simulink model "Roteiro1_Planta"  (R2019a)
settings: Solver=FixedStepAuto  StartTime=0.0  StopTime=250  FixedStep=0.1  RelTol=1e-3
values from neighbouring files (symbols this model uses):
  K = 0.4725    [Roteiro1_PlantaTermica.m]
  Kp = T/(K*L)    (= 21.164021164)    [Roteiro1_PlantaTermica.m]
  L = 10    [Roteiro1_PlantaTermica.m]
  T = 100    [Roteiro1_PlantaTermica.m]
  theta_AMB = 33.6    [Roteiro1_PlantaTermica.m]
settings Model: Creator=JoaoG-PC  LastModifiedBy=JoaoG-PC

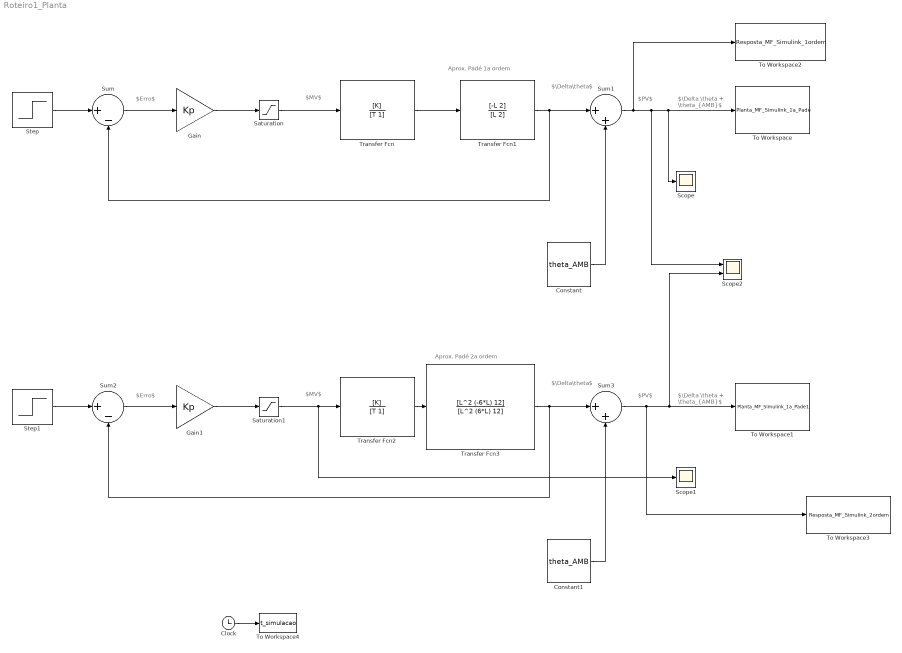
== system Roteiro1_Planta ==
  note: $Erro$
  note: $MV$
  note: Aprox. Padé 1a ordem
  note: $\Delta\theta$
  note: $PV$
  note: $\Delta \theta + \theta_{AMB}$
  note: $PV$
  note: $\Delta\theta$
  note: $Erro$
  note: $MV$
  note: $\Delta \theta + \theta_{AMB}$
  note: Aprox. Padé 2a ordem
  Clock : Clock
  Constant : Constant  Value=theta_AMB
  Constant1 : Constant  Value=theta_AMB
  Gain : Gain  Gain=Kp
  Gain1 : Gain  Gain=Kp
  Saturation : Saturate  UpperLimit=100  LowerLimit=0
  Saturation1 : Saturate  UpperLimit=100  LowerLimit=0
  Scope : Scope
  Scope1 : Scope
  Scope2 : Scope  NumInputPorts=2
  Step : Step  After=45-theta_AMB  SampleTime=0
  Step1 : Step  After=45-theta_AMB  SampleTime=0
  Sum : Sum  Inputs=|+-
  Sum1 : Sum  Inputs=|++
  Sum2 : Sum  Inputs=|+-
  Sum3 : Sum  Inputs=|++
  To Workspace : ToWorkspace  VariableName=Planta_MF_Simulink_1a_Pade  SampleTime=-1
  To Workspace1 : ToWorkspace  VariableName=Planta_MF_Simulink_1a_Pade1  SampleTime=-1
  To Workspace2 : ToWorkspace  VariableName=Resposta_MF_Simulink_1ordem  SampleTime=-1
  To Workspace3 : ToWorkspace  VariableName=Resposta_MF_Simulink_2ordem  SampleTime=-1
  To Workspace4 : ToWorkspace  VariableName=t_simulacao  SampleTime=-1
  Transfer Fcn : TransferFcn  Numerator=[K]  Denominator=[T 1]
  Transfer Fcn1 : TransferFcn  Numerator=[-L 2]  Denominator=[L 2]
  Transfer Fcn2 : TransferFcn  Numerator=[K]  Denominator=[T 1]
  Transfer Fcn3 : TransferFcn  Numerator=[L^2 (-6*L) 12]  Denominator=[L^2 (6*L) 12]
  wires:
  Transfer Fcn/1 -> Transfer Fcn1/1
  Transfer Fcn1/1 -> Sum1/1, Sum/2
  Sum/1 -> Gain/1
  Constant/1 -> Sum1/2
  Step/1 -> Sum/1
  Sum1/1 -> To Workspace2/1, Scope2/1, Scope/1, To Workspace/1
  Gain/1 -> Saturation/1
  Saturation/1 -> Transfer Fcn/1
  Saturation1/1 -> Scope1/1, Transfer Fcn2/1
  Gain1/1 -> Saturation1/1
  Constant1/1 -> Sum3/2
  Step1/1 -> Sum2/1
  Transfer Fcn3/1 -> Sum2/2, Sum3/1
  Transfer Fcn2/1 -> Transfer Fcn3/1
  Sum2/1 -> Gain1/1
  Sum3/1 -> To Workspace3/1, Scope2/2, To Workspace1/1
  Clock/1 -> To Workspace4/1
